simulink model "ADCS_MIL"  (R2024a)
settings: Solver=FixedStepAuto  StartTime=0.0  StopTime=6000  RelTol=1e-3
undefined symbols (not defined in the file or in its folder): agh, attitude, Cd, dgh, Eearth, epoch, Esun, Jsc, juliandate, k_Bdot, Kd1, Kd2, Kd3, km, Kp1, Kp2, Kp3, m, m_disturb, MTQ_Swithces, NoiseStd, s, satellite, signQuat, simulator, Surf_areas, Surf_dist, Surf_normals, Surf_reflectivity, WMM2020
libraries: sharedtransform x18, aerolibconvert2 x12, SepehrMILLib x11, simulink_extras x8, aerolibsatdyn x5, aerolibutil x5, sharedutil x3, vrlib x3, aerolibtransform2 x3, aerolibgravity2 x3, matrix_library x2
(part 2 of 3)

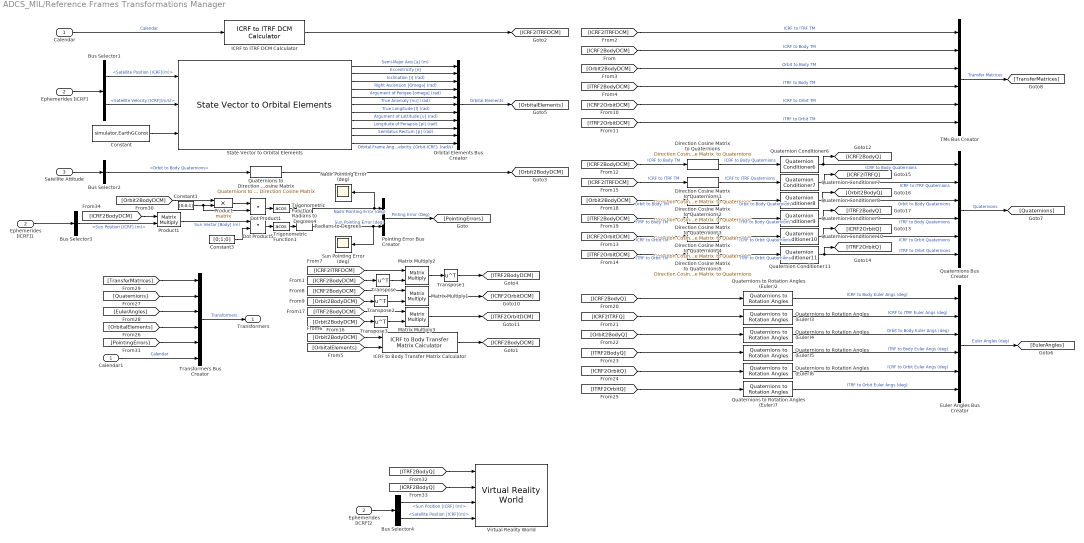
== system ADCS_MIL/Reference Frames Transformations Manager ==
  Calendar : Inport
  Ephemerides [ICRF] : Inport  Port=2
  Satellite Attitude : Inport  Port=3
  Bus Selector1 : BusSelector  OutputSignals=Satellite Ephemeris [ICRF].Satellite Position [ICRF](m),Satellite Ephemeris [ICRF].Satellite Velocity [ICRF](m/s)
  Bus Selector2 : BusSelector  OutputSignals=Orbit to Body Quaternions
  Bus Selector3 : BusSelector  OutputSignals=Sun Ephemeris [ICRF].Sun Position [ICRF] (m)
  Bus Selector4 : BusSelector  OutputSignals=Sun Ephemeris [ICRF].Sun Position [ICRF] (m),Satellite Ephemeris [ICRF].Satellite Position [ICRF](m)
  Calendar1 : InportShadow
  Constant : Constant  Value=simulator.EarthGConst
  Constant1 : Constant  Value=[0;0;1]
  Constant3 : Constant  Value=[0;1;0]
  Direction Cosine Matrix to Quaternions{,1..5} (6 alike) : sharedtransform/Direction Cosine Matrix  to Quaternions  aMode=0  action=None  tolerance=eps(2)
  Dot Product1 : DotProduct  OutDataTypeStr=Inherit: Inherit via internal rule
  Dot Product5 : DotProduct  OutDataTypeStr=Inherit: Inherit via internal rule
  Ephemerides [ICRF]1 : InportShadow  Port=2
  Ephemerides [ICRF]2 : InportShadow  Port=2
  Euler Angles Bus Creator : BusCreator  Inputs=6
  ICRF to Body Transfer Matrix Calculator : SepehrMILLib/Reference Frames Transformations Manager/ICRF to Body Transfer Matrix Calculator  SystemSampleTime=-1  VariantActivationTime=update diagram  AllowFlexibleInterface=on  Latency=0  AutoFrameSizeCalculation=off
  ICRF to ITRF DCM Calculator : SepehrMILLib/Reference Frames Transformations Manager/ICRF to ITRF DCM Calculator  SystemSampleTime=-1  VariantActivationTime=update diagram  AllowFlexibleInterface=on  Latency=0  AutoFrameSizeCalculation=off
  Matrix Multiply1 : Product  Multiplication=Matrix(*)
  Matrix Multiply2 : Product  Multiplication=Matrix(*)
  Matrix Multiply3 : Product  Multiplication=Matrix(*)
  Nadir Pointing Error (deg) : Scope
  Orbital Elements Bus Creator : BusCreator  Inputs=11
  Pointing Error Bus Creator : BusCreator  Inputs=2
  Product : Product  Multiplication=Matrix(*)
  Product1 : Product  Multiplication=Matrix(*)
  Quaternion Conditioner10 : SepehrMILLib/Reference Frames Transformations Manager/Quaternion Conditioner10  SystemSampleTime=-1  VariantActivationTime=update diagram  AllowFlexibleInterface=on  Latency=0  AutoFrameSizeCalculation=off
  Quaternion Conditioner11 : SepehrMILLib/Reference Frames Transformations Manager/Quaternion Conditioner11  SystemSampleTime=-1  VariantActivationTime=update diagram  AllowFlexibleInterface=on  Latency=0  AutoFrameSizeCalculation=off
  Quaternion Conditioner6 : SepehrMILLib/Reference Frames Transformations Manager/Quaternion Conditioner6  SystemSampleTime=-1  VariantActivationTime=update diagram  AllowFlexibleInterface=on  Latency=0  AutoFrameSizeCalculation=off
  Quaternion Conditioner7 : SepehrMILLib/Reference Frames Transformations Manager/Quaternion Conditioner7  SystemSampleTime=-1  VariantActivationTime=update diagram  AllowFlexibleInterface=on  Latency=0  AutoFrameSizeCalculation=off
  Quaternion Conditioner8 : SepehrMILLib/Reference Frames Transformations Manager/Quaternion Conditioner8  SystemSampleTime=-1  VariantActivationTime=update diagram  AllowFlexibleInterface=on  Latency=0  AutoFrameSizeCalculation=off
  Quaternion Conditioner9 : SepehrMILLib/Reference Frames Transformations Manager/Quaternion Conditioner9  SystemSampleTime=-1  VariantActivationTime=update diagram  AllowFlexibleInterface=on  Latency=0  AutoFrameSizeCalculation=off
  Quaternions Bus Creator : BusCreator  Inputs=6
  Quaternions to Direction Cosine Matrix : sharedtransform/Quaternions to  Direction Cosine Matrix  aMode=aMode
  Quaternions to Rotation Angles (Euler){2..7} (6 alike) : sharedtransform/Quaternions to Rotation Angles  rotationOrder=XYZ  aMode=aMode
  Radians to Degrees : simulink_extras/Transformations/Radians to Degrees
  Radians to Degrees4 : simulink_extras/Transformations/Radians to Degrees
  State Vector to Orbital Elements : SepehrMILLib/Reference Frames Transformations Manager/State Vector to Orbital Elements  SystemSampleTime=-1  VariantActivationTime=update diagram  AllowFlexibleInterface=on  Latency=0  AutoFrameSizeCalculation=off
  Sun Pointing Error (deg) : Scope
  TMs Bus Creator : BusCreator  Inputs=6
  Transformers Bus Creator : BusCreator  Inputs=6
  Transpose{,1..3} (4 alike) : Math  Operator=transpose
  Trigonometric Function : Trigonometry  Operator=acos
  Trigonometric Function1 : Trigonometry  Operator=acos  OutputSignalType=real
  Virtual Reality World : SepehrMILLib/Reference Frames Transformations Manager/Virtual Reality World  SystemSampleTime=-1  VariantControl=visSL3D  VariantActivationTime=update diagram  AllowFlexibleInterface=on  Latency=0  AutoFrameSizeCalculation=off
  Transformers : Outport
  wires:
  State Vector to Orbital Elements/7 -> Orbital Elements Bus Creator/7  "True Longitude [l] (rad)"
  Quaternion Conditioner8/1 -> Quaternions Bus Creator/3, [Orbit2BodyQ]  "Orbit to Body Quaternions"
  [Orbit2BodyQ] -> Quaternions to Rotation Angles (Euler)4/1
  [ITRF2OrbitQ] -> Quaternions to Rotation Angles (Euler)7/1
  [ITRF2OrbitDCM] -> Direction Cosine Matrix to Quaternions5/1  "ITRF to Orbit TM"
  Bus Selector1/2 -> State Vector to Orbital Elements/2  "<Satellite Velocity [ICRF](m/s)>"
  [ICRF2ITRFQ] -> Quaternions to Rotation Angles (Euler)3/1
  [Orbit2BodyDCM] -> Transpose3/1
  [ICRF2OrbitQ] -> Quaternions to Rotation Angles (Euler)6/1
  [ICRF2BodyDCM] -> Matrix Multiply1/1
  [EulerAngles] -> Transformers Bus Creator/3
  State Vector to Orbital Elements/6 -> Orbital Elements Bus Creator/6  "True Anomaly [nu] (rad)"
  State Vector to Orbital Elements/5 -> Orbital Elements Bus Creator/5  "Argument of Perigee [omega] (rad)"
  Bus Selector4/1 -> Virtual Reality World/3  "<Sun Position [ICRF] (m)>"
  Transformers Bus Creator/1 -> Transformers/1  "Transformers"
  State Vector to Orbital Elements/4 -> Orbital Elements Bus Creator/4  "Right Ascension [Omega] (rad)"
  State Vector to Orbital Elements/10 -> Orbital Elements Bus Creator/10  "Semilatus Rectum [p] (rad)"
  State Vector to Orbital Elements/9 -> Orbital Elements Bus Creator/9  "Longitude of Periapsis [pi] (rad)"
  Quaternion Conditioner10/1 -> Quaternions Bus Creator/5, [ICRF2OrbitQ]  "ICRF to Orbit Quaternions"
  State Vector to Orbital Elements/8 -> Orbital Elements Bus Creator/8  "Argument of Lattitude [u] (rad)"
  Quaternions to Direction Cosine Matrix/1 -> [Orbit2BodyDCM]
  State Vector to Orbital Elements/1 -> Orbital Elements Bus Creator/1  "Semi-Major Axis [a] (m)"
  [OrbitalElements] -> ICRF to Body Transfer Matrix Calculator/2
  Ephemerides [ICRF]1/1 -> Bus Selector3/1
  Dot Product5/1 -> Trigonometric Function1/1
  [ICRF2BodyDCM] -> Transpose/1
  Matrix Multiply2/1 -> Transpose1/1
  [ITRF2BodyQ] -> Virtual Reality World/1
  Bus Selector1/1 -> State Vector to Orbital Elements/1  "<Satellite Position [ICRF](m)>"
  ICRF to Body Transfer Matrix Calculator/1 -> [ICRF2BodyDCM]
  Transpose2/1 -> Matrix Multiply1/2
  ICRF to ITRF DCM Calculator/1 -> [ICRF2ITRFDCM]
  Orbital Elements Bus Creator/1 -> [OrbitalElements]  "Orbital Elements"
  Transpose1/1 -> [ITRF2BodyDCM]
  Trigonometric Function/1 -> Radians to Degrees4/1
  Matrix Multiply3/1 -> [ITRF2OrbitDCM]
  Constant3/1 -> Dot Product5/2
  [OrbitalElements] -> Transformers Bus Creator/4
  [ITRF2BodyDCM] -> Matrix Multiply3/1
  Transpose3/1 -> Matrix Multiply3/2
  Radians to Degrees4/1 -> Pointing Error Bus Creator/1, Nadir Pointing Error (deg)/1  "Nadir Pointing Error (deg)"
  Radians to Degrees/1 -> Sun Pointing Error (deg)/1, Pointing Error Bus Creator/2  "Sun Pointing Error (deg)"
  Calendar/1 -> ICRF to ITRF DCM Calculator/1  "Calendar"
  Bus Selector4/2 -> Virtual Reality World/4  "<Satellite Position [ICRF](m)>"
  Pointing Error Bus Creator/1 -> [PointingErrors]  "Pinting Error (Deg)"
  [ICRF2BodyQ] -> Virtual Reality World/2
  State Vector to Orbital Elements/11 -> Orbital Elements Bus Creator/11  "Orbital Frame Angular Velocity {Orbit-ICRF} (rad/s)"
  Constant/1 -> State Vector to Orbital Elements/3
  [Orbit2BodyDCM] -> Direction Cosine Matrix to Quaternions2/1  "Orbit to Body TM"
  [ICRF2ITRFDCM] -> TMs Bus Creator/1  "ICRF to ITRF TM"
  [ICRF2BodyDCM] -> TMs Bus Creator/2  "ICRF to Body TM"
  [PointingErrors] -> Transformers Bus Creator/5
  Transpose/1 -> Matrix Multiply2/2
  [Orbit2BodyDCM] -> Product/1
  Direction Cosine Matrix to Quaternions/1 -> Quaternion Conditioner6/1  "ICRF to Body Quaternions"
  [ICRF2OrbitDCM] -> TMs Bus Creator/5  "ICRF to Orbit TM"
  Quaternion Conditioner11/1 -> Quaternions Bus Creator/6, [ITRF2OrbitQ]  "ITRF to Orbit Quaternions"
  Direction Cosine Matrix to Quaternions3/1 -> Quaternion Conditioner9/1  "ITRF to Body Quaternions"
  [ICRF2BodyQ] -> Quaternions to Rotation Angles (Euler)2/1
  Constant1/1 -> Product/2, Dot Product1/2
  [ITRF2BodyDCM] -> TMs Bus Creator/4  "ITRF to Body TM"
  Quaternions to Rotation Angles (Euler)7/1 -> Euler Angles Bus Creator/6  "ITRF to Orbit Euler Angs (deg)"
  [Quaternions] -> Transformers Bus Creator/2
  [ITRF2OrbitDCM] -> TMs Bus Creator/6  "ITRF to Orbit TM"
  [ICRF2ITRFDCM] -> Matrix Multiply2/1
  Satellite Attitude/1 -> Bus Selector2/1
  Calendar1/1 -> Transformers Bus Creator/6  "Calendar"
  State Vector to Orbital Elements/2 -> Orbital Elements Bus Creator/2  "Eccentricity [e]"
  Quaternion Conditioner7/1 -> Quaternions Bus Creator/2, [ICRF2ITRFQ]  "ICRF to ITRF Quaternions"
  Ephemerides [ICRF]/1 -> Bus Selector1/1
  Quaternions Bus Creator/1 -> [Quaternions]  "Quaternions"
  [ICRF2ITRFDCM] -> Direction Cosine Matrix to Quaternions1/1  "ICRF to ITRF TM"
  Matrix Multiply1/1 -> [ICRF2OrbitDCM]
  Ephemerides [ICRF]2/1 -> Bus Selector4/1
  Direction Cosine Matrix to Quaternions5/1 -> Quaternion Conditioner11/1  "ITRF to Orbit Quaternions"
  Direction Cosine Matrix to Quaternions4/1 -> Quaternion Conditioner10/1  "ICRF to Orbit Quaternions"
  TMs Bus Creator/1 -> [TransferMatrices]  "Transfer Matrices"
  [ITRF2BodyDCM] -> Direction Cosine Matrix to Quaternions3/1  "ITRF to Body TM"
  Product1/1 -> Dot Product5/1  "Sun Vector [Body] (m)"
  Product/1 -> Dot Product1/1
  Bus Selector2/1 -> Quaternions to Direction Cosine Matrix/1  "<Orbit to Body Quaternions>"
  [Orbit2BodyDCM] -> Transpose2/1
  Quaternion Conditioner9/1 -> Quaternions Bus Creator/4, [ITRF2BodyQ]  "ITRF to Body Quaternions"
  Direction Cosine Matrix to Quaternions2/1 -> Quaternion Conditioner8/1  "Orbit to Body Quaternions"
  Quaternion Conditioner6/1 -> Quaternions Bus Creator/1, [ICRF2BodyQ]  "ICRF to Body Quaternions"
  Quaternions to Rotation Angles (Euler)5/1 -> Euler Angles Bus Creator/4  "ITRF to Body Euler Angs (deg)"
  Dot Product1/1 -> Trigonometric Function/1
  Direction Cosine Matrix to Quaternions1/1 -> Quaternion Conditioner7/1  "ICRF to ITRF Quaternions"
  Quaternions to Rotation Angles (Euler)2/1 -> Euler Angles Bus Creator/1  "ICRF to Body Euler Angs (deg)"
  Quaternions to Rotation Angles (Euler)3/1 -> Euler Angles Bus Creator/2  "ICRF to ITRF Euler Angs (deg)"
  Euler Angles Bus Creator/1 -> [EulerAngles]  "Euler Angles (deg)"
  State Vector to Orbital Elements/3 -> Orbital Elements Bus Creator/3  "Inclination [i] (rad)"
  [TransferMatrices] -> Transformers Bus Creator/1
  [ICRF2OrbitDCM] -> Direction Cosine Matrix to Quaternions4/1  "ICRF to Orbit TM"
  Quaternions to Rotation Angles (Euler)6/1 -> Euler Angles Bus Creator/5  "ICRF to Orbit Euler Angs (deg)"
  [ITRF2BodyQ] -> Quaternions to Rotation Angles (Euler)5/1
  [Orbit2BodyDCM] -> TMs Bus Creator/3  "Orbit to Body TM"
  Trigonometric Function1/1 -> Radians to Degrees/1
  Quaternions to Rotation Angles (Euler)4/1 -> Euler Angles Bus Creator/3  "Orbit to Body Euler Angs (deg)"
  [ICRF2BodyDCM] -> Direction Cosine Matrix to Quaternions/1  "ICRF to Body TM"
  [Orbit2BodyDCM] -> ICRF to Body Transfer Matrix Calculator/1
  [ICRF2BodyDCM] -> Product1/1
  Bus Selector3/1 -> Product1/2  "<Sun Position [ICRF] (m)>"

== system ADCS_MIL/Satellite Position [ICRF2ITRF] ==
  Satellite Position [ICRF] : Inport
  Onboard Calendar : Inport  Port=2
  Bus Selector : BusSelector  OutputSignals=Onboard Satellite Position [ICRF] (m)
  ICRF to ITRF DCM Calculator : SepehrMILLib/Reference Frames Transformations Manager/ICRF to ITRF DCM Calculator  SystemSampleTime=-1  VariantActivationTime=update diagram  AllowFlexibleInterface=on  Latency=0  AutoFrameSizeCalculation=off
  Product1 : Product  Multiplication=Matrix(*)
  Satellite Position [ITRF] (m) : Outport
  wires:
  ICRF to ITRF DCM Calculator/1 -> [ICRF2ITRFDCM]
  Onboard Calendar/1 -> ICRF to ITRF DCM Calculator/1  "Calendar"
  [ICRF2ITRFDCM] -> Product1/1
  Satellite Position [ICRF]/1 -> Bus Selector/1
  Product1/1 -> Satellite Position [ITRF] (m)/1  "Onboard_Satellite Position [ITRF] (m)"
  Bus Selector/1 -> Product1/2  "<Onboard Satellite Position [ICRF] (m)>"

== system ADCS_MIL/Sensors ==
  Calendar : Inport
  Satellite Ephemeris : Inport  Port=2
  Satellite Attitude : Inport  Port=3
  Sensor Switch : Inport  Port=4
  MM_Temp : Inport  Port=5
  Measurement Model DCM : Inport  Port=6
  Eclipse : Inport  Port=7
  Input Voltage(V) : Inport  Port=8
  B_Body : Inport  Port=9
  Sun Ephemeris [ICRF] : Inport  Port=10
  Transformers : Inport  Port=11
  Bus Creator : BusCreator  Inputs=3
  Bus Selector : BusSelector  OutputSignals=Angular Velocity {Body-ICRF}(rad/s)
  Bus Selector1 : BusSelector  OutputSignals=Sun Position [ICRF] (m)
  Bus Selector2 : BusSelector  OutputSignals=Quaternions.ICRF to Body Quaternions
  GNSS Receiver Model : Subsystem
  Gyroscope Model : Subsystem
  Magnetometer Model : Subsystem
  Sun Sensor Model : Subsystem
  Sun Position Measured [Body] : Outport
  B Measured [Body] : Outport  Port=2
  Angular Velocity Measured [Body] : Outport  Port=3
  Satellite Measured Ephemeris : Outport  Port=4
  Current (A) : Outport  Port=5
  wires:
  Calendar/1 -> GNSS Receiver Model/1(Calendar)
  Satellite Ephemeris/1 -> GNSS Receiver Model/2(Satellite Ephemeris)
  Satellite Attitude/1 -> Bus Selector/1
  Sensor Switch/1 -> Magnetometer Model/5(Sensor Switch), GNSS Receiver Model/4(Sensor Switch), Gyroscope Model/4(Sensor Switch)
  MM_Temp/1 -> Magnetometer Model/2(Temperature (˚C))
  Input Voltage(V)/1 -> Magnetometer Model/3(Input Voltage (V)), GNSS Receiver Model/3(" Input Voltage (V)"), Gyroscope Model/2(Input Voltage (V))
  Measurement Model DCM/1 -> Gyroscope Model/3(Measurement Model DCM), Magnetometer Model/4(Measurement Model DCM)
  Eclipse/1 -> Sun Sensor Model/1(Eclipse)
  Sun Sensor Model/1(SunPos_Sensed(Body)) -> Sun Position Measured [Body]/1
  Magnetometer Model/2(Power (W)) -> Bus Creator/3  "Magnetometer Power (W)"
  Magnetometer Model/1(Magnetic Field [Sensor](T)) -> B Measured [Body]/1
  Gyroscope Model/2(Power (W)) -> Bus Creator/2  "Gyro Power (W)"
  GNSS Receiver Model/2(Power (W)) -> Bus Creator/1  "Power GNSS Receiver (W)"
  Bus Creator/1 -> Current (A)/1
  GNSS Receiver Model/1(Measured Satellite Ephemeris) -> Satellite Measured Ephemeris/1
  Gyroscope Model/1(Measured Angular Velocity [Sensor] (rad/s)) -> Angular Velocity Measured [Body]/1
  B_Body/1 -> Magnetometer Model/1(Magnetic Field [Body] (T))
  Bus Selector/1 -> Gyroscope Model/1(Angular Velocity [Body] (rad/s))  "<Angular Velocity {Body-ICRF}(rad/s)>"
  Sun Ephemeris [ICRF]/1 -> Bus Selector1/1
  Bus Selector1/1 -> Sun Sensor Model/3(SunPos[ICRF])  "<Sun Position [ICRF] (m)>"
  Transformers/1 -> Bus Selector2/1
  Bus Selector2/1 -> Sun Sensor Model/2(q[ICRFtoBody])  "<ICRF to Body Quaternions>"

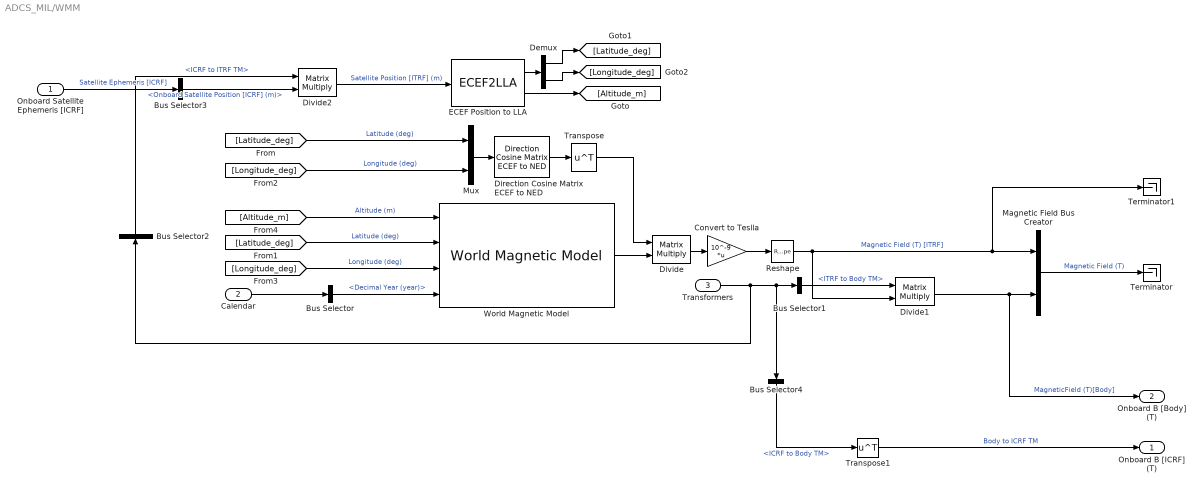
== system ADCS_MIL/WMM ==
  Onboard Satellite Ephemeris [ICRF] : Inport
  Calendar : Inport  Port=2
  Transformers : Inport  Port=3
  Bus Selector : BusSelector  OutputSignals=Decimal Year (year)
  Bus Selector1 : BusSelector  OutputSignals=Transfer Matrices.ITRF to Body TM
  Bus Selector2 : BusSelector  OutputSignals=Transfer Matrices.ICRF to ITRF TM
  Bus Selector3 : BusSelector  OutputSignals=Onboard Satellite Position [ICRF] (m)
  Bus Selector4 : BusSelector  OutputSignals=Transfer Matrices.ICRF to Body TM
  Convert to Teslla : Gain  Gain=10^-9  Multiplication=Matrix(K*u)
  Demux : Demux  Outputs=2
  Direction Cosine Matrix ECEF to NED : aerolibtransform2/Direction Cosine Matrix ECEF to NED
  Divide : Product  Inputs=**  Multiplication=Matrix(*)
  Divide1 : Product  Inputs=**  Multiplication=Matrix(*)
  Divide2 : Product  Inputs=**  Multiplication=Matrix(*)
  ECEF Position to LLA : ECEF2LLA
  Magnetic Field Bus Creator : BusCreator  Inputs=2
  Mux : Mux  Inputs=2
  Reshape : Reshape  OutputDimensionality=Customize  OutputDimensions=[3,1]
  Terminator : Terminator
  Terminator1 : Terminator
  Transpose : Math  Operator=transpose
  Transpose1 : Math  Operator=transpose
  World Magnetic Model : aerolibgravity2/World Magnetic Model  model=WMM2020 (2020-2025)  customFile='WMM2020.COF'  units=Metric (MKS)  time_in=on  month=January  day=1  year=2020  action=Error  h_out=off  dec_out=off  inc_out=off  ti_out=off
  Onboard B [ICRF] (T) : Outport
  Onboard B [Body] (T) : Outport  Port=2
  wires:
  [Latitude_deg] -> World Magnetic Model/2  "Latitude (deg)"
  Transpose/1 -> Divide/1
  Demux/1 -> [Latitude_deg]
  [Altitude_m] -> World Magnetic Model/1  "Altitude (m)"
  Reshape/1 -> Terminator1/1, Magnetic Field Bus Creator/1, Divide1/2  "Magnetic Field (T) [ITRF]"
  Direction Cosine Matrix ECEF to NED/1 -> Transpose/1
  Magnetic Field Bus Creator/1 -> Terminator/1  "Magnetic Field (T)"
  Mux/1 -> Direction Cosine Matrix ECEF to NED/1
  Transformers/1 -> Bus Selector1/1, Bus Selector4/1, Bus Selector2/1
  [Latitude_deg] -> Mux/1  "Latitude (deg)"
  [Longitude_deg] -> Mux/2  "Longitude (deg)"
  ECEF Position to LLA/2 -> [Altitude_m]
  Demux/2 -> [Longitude_deg]
  Divide/1 -> Convert to Teslla/1
  Convert to Teslla/1 -> Reshape/1
  Calendar/1 -> Bus Selector/1
  ECEF Position to LLA/1 -> Demux/1
  Divide2/1 -> ECEF Position to LLA/1  "Satellite Position [ITRF] (m)"
  [Longitude_deg] -> World Magnetic Model/3  "Longitude (deg)"
  Bus Selector/1 -> World Magnetic Model/4  "<Decimal Year (year)>"
  Divide1/1 -> Onboard B [Body] (T)/1, Magnetic Field Bus Creator/2  "MagneticField (T)[Body]"
  World Magnetic Model/1 -> Divide/2
  Bus Selector1/1 -> Divide1/1  "<ITRF to Body TM>"
  Onboard Satellite Ephemeris [ICRF]/1 -> Bus Selector3/1  "Satellite Ephemeris [ICRF]"
  Bus Selector2/1 -> Divide2/1  "<ICRF to ITRF TM>"
  Bus Selector3/1 -> Divide2/2  "<Onboard Satellite Position [ICRF] (m)>"
  Bus Selector4/1 -> Transpose1/1  "<ICRF to Body TM>"
  Transpose1/1 -> Onboard B [ICRF] (T)/1  "Body to ICRF TM"

== system ADCS_MIL/Attitude Controlgg/On.Nadir_Pointing/Nadir Pointing ==
  Ephemeris : Inport
  q(body2ICRF) : Inport  Port=2
  Omega(Body) : Inport  Port=3
  B(Body) : Inport  Port=4
  Kd : Constant  Value=[1 1 1]
  Kp : Constant  Value=[1 1 1]
  PD Controller : Subsystem
  q_Desired Propagator : Subsystem
  q_error Calculator : Subsystem
  m_Command : Outport
  wires:
  q(body2ICRF)/1 -> q_error Calculator/2(q_Real)
  Ephemeris/1 -> q_Desired Propagator/1(Ephemeris)
  q_Desired Propagator/1(q_Desired) -> q_error Calculator/1(q_Desired)
  PD Controller/1(m_Command) -> m_Command/1
  q_error Calculator/1(q_error) -> PD Controller/3(q_Error)
  Kp/1 -> PD Controller/4(Kp)
  Kd/1 -> PD Controller/5(Kd)
  Omega(Body)/1 -> PD Controller/1(Omega(Body))
  B(Body)/1 -> PD Controller/2(B(Body))

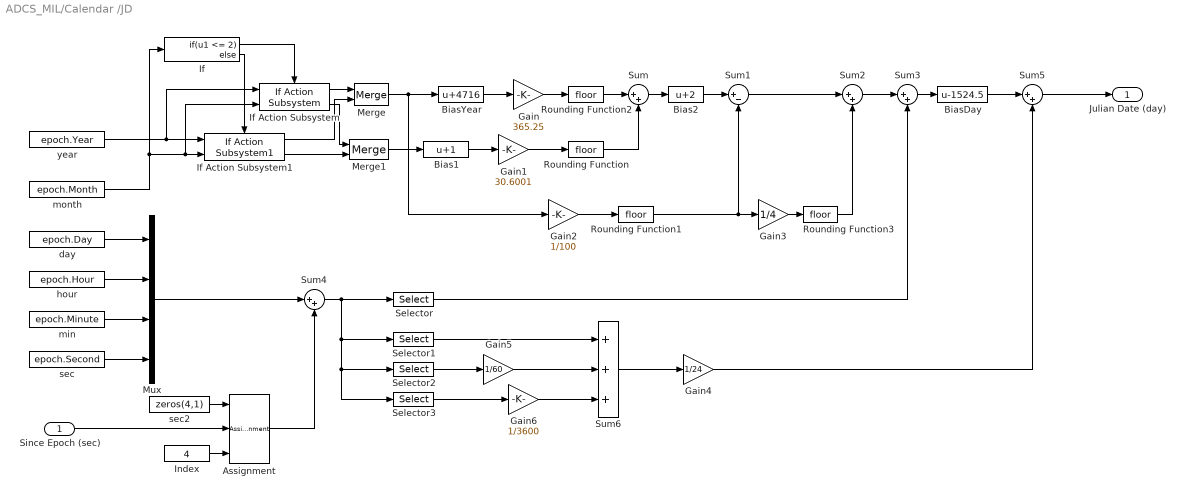
== system ADCS_MIL/Calendar /JD ==
  Since Epoch (sec) : Inport  OutMin=0  PortDimensions=1
  Assignment : Assignment  IndexOptions=Index vector (port)  Indices=1  OutputSizes=1
  Bias1 : Bias  Bias=1  SaturateOnIntegerOverflow=off
  Bias2 : Bias  Bias=2  SaturateOnIntegerOverflow=off
  BiasDay : Bias  Bias=-1524.5  SaturateOnIntegerOverflow=off
  BiasYear : Bias  Bias=4716  SaturateOnIntegerOverflow=off
  Gain : Gain  Gain=365.25
  Gain1 : Gain  Gain=30.6001
  Gain2 : Gain  Gain=1/100
  Gain3 : Gain  Gain=1/4
  Gain4 : Gain  Gain=1/24
  Gain5 : Gain  Gain=1/60
  Gain6 : Gain  Gain=1/3600
  If : If  IfExpression=u1 <= 2
  If Action Subsystem : aerolibconvert2/Julian Date Conversion/If Action Subsystem  SystemSampleTime=-1  VariantActivationTime=update diagram  AllowFlexibleInterface=on  Latency=0  AutoFrameSizeCalculation=off
  If Action Subsystem1 : aerolibconvert2/Julian Date Conversion/If Action Subsystem1  SystemSampleTime=-1  VariantActivationTime=update diagram  AllowFlexibleInterface=on  Latency=0  AutoFrameSizeCalculation=off
  Index : Constant  Value=4
  Merge : Merge
  Merge1 : Merge
  Mux : Mux
  Rounding Function{,1..3} (4 alike) : Rounding
  Selector : Selector  InputPortWidth=4  IndexOptions=Index vector (dialog)  Indices=[1]  OutputSizes=1
  Selector1 : Selector  InputPortWidth=4  IndexOptions=Index vector (dialog)  Indices=[2]  OutputSizes=1
  Selector2 : Selector  InputPortWidth=4  IndexOptions=Index vector (dialog)  Indices=[3]  OutputSizes=1
  Selector3 : Selector  InputPortWidth=4  IndexOptions=Index vector (dialog)  Indices=[4]  OutputSizes=1
  Sum{,2..5} (5 alike) : Sum  Inputs=|++
  Sum1 : Sum  Inputs=|+-
  Sum6 : Sum  Inputs=+++
  day : Constant  Value=epoch.Day
  hour : Constant  Value=epoch.Hour
  min : Constant  Value=epoch.Minute
  month : Constant  Value=epoch.Month
  sec : Constant  Value=epoch.Second
  sec2 : Constant  Value=zeros(4,1)
  year : Constant  Value=epoch.Year
  Julian Date (day) : Outport  VectorParamsAs1DForOutWhenUnconnected=off
  wires:
  Merge1/1 -> Bias1/1
  Mux/1 -> Sum4/1
  month/1 -> If/1, If Action Subsystem1/2, If Action Subsystem/2
  Rounding Function/1 -> Sum/2
  day/1 -> Mux/1
  If Action Subsystem1/2 -> Merge1/2
  Sum/1 -> Bias2/1
  Sum6/1 -> Gain4/1
  BiasDay/1 -> Sum5/1
  hour/1 -> Mux/2
  Selector/1 -> Sum3/2
  sec/1 -> Mux/4
  Since Epoch (sec)/1 -> Assignment/2
  If/2 -> If Action Subsystem1/Action
  Rounding Function1/1 -> Sum1/2, Gain3/1
  Gain5/1 -> Sum6/2
  Assignment/1 -> Sum4/2
  Bias2/1 -> Sum1/1
  Gain/1 -> Rounding Function2/1
  Gain2/1 -> Rounding Function1/1
  Sum4/1 -> Selector/1, Selector3/1, Selector2/1, Selector1/1
  If Action Subsystem/1 -> Merge/1
  year/1 -> If Action Subsystem1/1, If Action Subsystem/1
  Gain6/1 -> Sum6/3
  Sum3/1 -> BiasDay/1
  If Action Subsystem/2 -> Merge1/1
  Bias1/1 -> Gain1/1
  Rounding Function3/1 -> Sum2/2
  Gain1/1 -> Rounding Function/1
  sec2/1 -> Assignment/1
  Sum1/1 -> Sum2/1
  Sum5/1 -> Julian Date (day)/1
  Selector1/1 -> Sum6/1
  Sum2/1 -> Sum3/1
  Gain4/1 -> Sum5/2
  BiasYear/1 -> Gain/1
  Merge/1 -> BiasYear/1, Gain2/1
  Gain3/1 -> Rounding Function3/1
  Selector2/1 -> Gain5/1
  Rounding Function2/1 -> Sum/1
  Selector3/1 -> Gain6/1
  If/1 -> If Action Subsystem/Action
  min/1 -> Mux/3
  If Action Subsystem1/1 -> Merge/2
  Index/1 -> Assignment/3

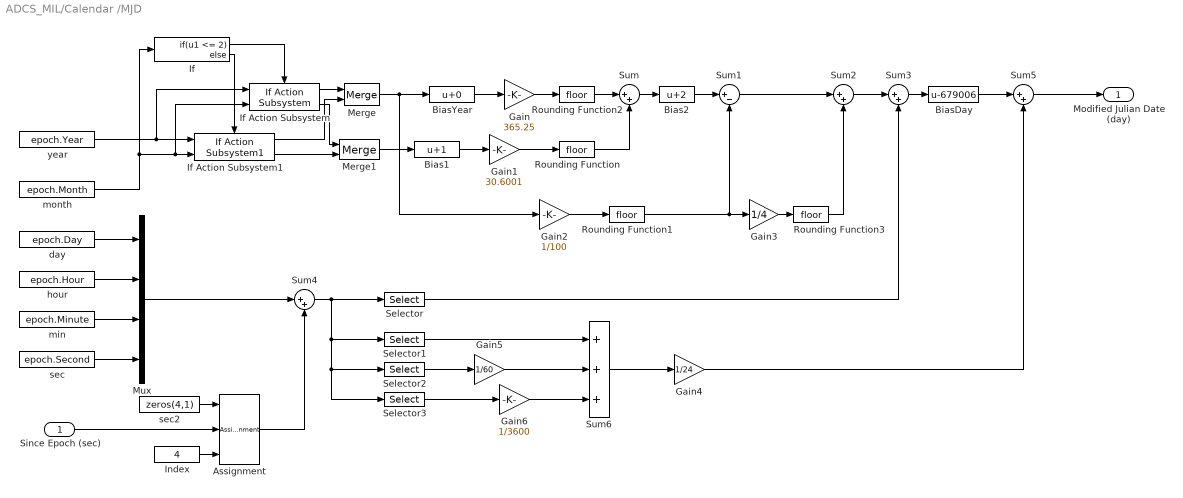
== system ADCS_MIL/Calendar /MJD ==
  Since Epoch (sec) : Inport  OutMin=0  PortDimensions=1
  Assignment : Assignment  IndexOptions=Index vector (port)  Indices=1  OutputSizes=1
  Bias1 : Bias  Bias=1  SaturateOnIntegerOverflow=off
  Bias2 : Bias  Bias=2  SaturateOnIntegerOverflow=off
  BiasDay : Bias  Bias=-679006  SaturateOnIntegerOverflow=off
  BiasYear : Bias  SaturateOnIntegerOverflow=off
  Gain : Gain  Gain=365.25
  Gain1 : Gain  Gain=30.6001
  Gain2 : Gain  Gain=1/100
  Gain3 : Gain  Gain=1/4
  Gain4 : Gain  Gain=1/24
  Gain5 : Gain  Gain=1/60
  Gain6 : Gain  Gain=1/3600
  If : If  IfExpression=u1 <= 2
  If Action Subsystem : aerolibconvert2/Julian Date Conversion/If Action Subsystem  SystemSampleTime=-1  VariantActivationTime=update diagram  AllowFlexibleInterface=on  Latency=0  AutoFrameSizeCalculation=off
  If Action Subsystem1 : aerolibconvert2/Julian Date Conversion/If Action Subsystem1  SystemSampleTime=-1  VariantActivationTime=update diagram  AllowFlexibleInterface=on  Latency=0  AutoFrameSizeCalculation=off
  Index : Constant  Value=4
  Merge : Merge
  Merge1 : Merge
  Mux : Mux
  Rounding Function{,1..3} (4 alike) : Rounding
  Selector : Selector  InputPortWidth=4  IndexOptions=Index vector (dialog)  Indices=[1]  OutputSizes=1
  Selector1 : Selector  InputPortWidth=4  IndexOptions=Index vector (dialog)  Indices=[2]  OutputSizes=1
  Selector2 : Selector  InputPortWidth=4  IndexOptions=Index vector (dialog)  Indices=[3]  OutputSizes=1
  Selector3 : Selector  InputPortWidth=4  IndexOptions=Index vector (dialog)  Indices=[4]  OutputSizes=1
  Sum{,2..5} (5 alike) : Sum  Inputs=|++
  Sum1 : Sum  Inputs=|+-
  Sum6 : Sum  Inputs=+++
  day : Constant  Value=epoch.Day
  hour : Constant  Value=epoch.Hour
  min : Constant  Value=epoch.Minute
  month : Constant  Value=epoch.Month
  sec : Constant  Value=epoch.Second
  sec2 : Constant  Value=zeros(4,1)
  year : Constant  Value=epoch.Year
  Modified Julian Date (day) : Outport  VectorParamsAs1DForOutWhenUnconnected=off
  wires:
  Rounding Function/1 -> Sum/2
  If/2 -> If Action Subsystem1/Action
  Gain4/1 -> Sum5/2
  BiasYear/1 -> Gain/1
  Bias2/1 -> Sum1/1
  Selector1/1 -> Sum6/1
  Sum/1 -> Bias2/1
  Sum2/1 -> Sum3/1
  BiasDay/1 -> Sum5/1
  Selector/1 -> Sum3/2
  Sum1/1 -> Sum2/1
  year/1 -> If Action Subsystem1/1, If Action Subsystem/1
  Sum5/1 -> Modified Julian Date (day)/1
  Sum6/1 -> Gain4/1
  hour/1 -> Mux/2
  Gain/1 -> Rounding Function2/1
  Merge1/1 -> Bias1/1
  Since Epoch (sec)/1 -> Assignment/2
  Gain6/1 -> Sum6/3
  Gain2/1 -> Rounding Function1/1
  Mux/1 -> Sum4/1
  Rounding Function1/1 -> Sum1/2, Gain3/1
  Rounding Function3/1 -> Sum2/2
  Sum3/1 -> BiasDay/1
  Selector3/1 -> Gain6/1
  Rounding Function2/1 -> Sum/1
  Gain1/1 -> Rounding Function/1
  sec2/1 -> Assignment/1
  day/1 -> Mux/1
  Bias1/1 -> Gain1/1
  min/1 -> Mux/3
  Gain3/1 -> Rounding Function3/1
  If/1 -> If Action Subsystem/Action
  Gain5/1 -> Sum6/2
  If Action Subsystem1/1 -> Merge/2
  Sum4/1 -> Selector/1, Selector3/1, Selector2/1, Selector1/1
  Merge/1 -> BiasYear/1, Gain2/1
  If Action Subsystem/1 -> Merge/1
  Selector2/1 -> Gain5/1
  If Action Subsystem/2 -> Merge1/1
  month/1 -> If/1, If Action Subsystem1/2, If Action Subsystem/2
  sec/1 -> Mux/4
  If Action Subsystem1/2 -> Merge1/2
  Assignment/1 -> Sum4/2
  Index/1 -> Assignment/3

== system ADCS_MIL/External Disturbance Torque/Drag ==
  Rsc_earth : Inport
  Vsc_earth : Inport  Port=2
  Abn : Inport  Port=3
  Constant : Constant  Value=Surf_normals
  Constant1 : Constant  Value=Surf_areas
  Constant2 : Constant  Value=Cd
  Constant4 : Constant  Value=Surf_dist
  MATLAB Function : MATLAB Function  TreatAsAtomicUnit=on
  Drag torque : Outport
  wires:
  Abn/1 -> MATLAB Function/3(Abn)
  Rsc_earth/1 -> MATLAB Function/1(Rearth)
  MATLAB Function/1(M_drag) -> Drag torque/1
  Constant/1 -> MATLAB Function/4(Surf_norms)
  Constant1/1 -> MATLAB Function/5(Surf_areas)
  Constant4/1 -> MATLAB Function/6(Surf_dist)
  Vsc_earth/1 -> MATLAB Function/2(Vearth)
  Constant2/1 -> MATLAB Function/7(Cd)

== system ADCS_MIL/External Disturbance Torque/Gravitional ==
  Rsc_earth : Inport
  Vsc_earth : Inport  Port=2
  Abn : Inport  Port=3
  Constant : Constant  Value=Jsc
  MATLAB Function : MATLAB Function  TreatAsAtomicUnit=on
  Grav torque : Outport
  wires:
  Abn/1 -> MATLAB Function/3(Abn)
  Rsc_earth/1 -> MATLAB Function/1(Rearth)
  MATLAB Function/1(M_grav) -> Grav torque/1
  Constant/1 -> MATLAB Function/4(J)
  Vsc_earth/1 -> MATLAB Function/2(Vearth)

== system ADCS_MIL/External Disturbance Torque/Magnetic ==
  Rsc_earth : Inport
  Earth RA : Inport  Port=2
  Abn : Inport  Port=3
  Att_req_inert1 : MATLAB Function  TreatAsAtomicUnit=on
  Constant : Constant  Value=agh
  Constant1 : Constant  Value=m_disturb
  Constant3 : Constant  Value=dgh
  Cross Product : vrlib/Utilities/Cross Product
  Magnetic Disturbance Torques Calculator : MATLAB Function  TreatAsAtomicUnit=on
  Product : Product  Multiplication=Matrix(*)
  Bn : Outport
  Bb : Outport  Port=2
  Magnetic torque : Outport  Port=3
  wires:
  Att_req_inert1/1(Bn) -> Product/2, Bn/1
  Rsc_earth/1 -> Att_req_inert1/3(R)
  Constant3/1 -> Att_req_inert1/1(dgh)
  Constant/1 -> Att_req_inert1/2(agh)
  Earth RA/1 -> Att_req_inert1/4(RA_earth_rot)
  Abn/1 -> Product/1
  Product/1 -> Cross Product/1, Bb/1
  Constant1/1 -> Cross Product/2
  Cross Product/1 -> Magnetic torque/1

== system ADCS_MIL/External Disturbance Torque/Radiation Pressure ==
  Rsc_sun : Inport
  Rsc_earth : Inport  Port=2
  Abn : Inport  Port=3
  Constant : Constant  Value=Surf_normals
  Constant1 : Constant  Value=Surf_areas
  Constant2 : Constant  Value=Surf_reflectivity
  Constant3 : Constant  Value=Esun
  Constant4 : Constant  Value=Surf_dist
  Constant5 : Constant  Value=Eearth
  MATLAB Function : MATLAB Function  TreatAsAtomicUnit=on
  MATLAB Function1 : MATLAB Function  TreatAsAtomicUnit=on
  Scope : Scope  NumInputPorts=2
  Sum : Sum
  RP torque : Outport
  wires:
  Abn/1 -> MATLAB Function1/2(Abn), MATLAB Function/2(Abn)
  Rsc_sun/1 -> MATLAB Function/1(Rsun)
  MATLAB Function/1(M_srp) -> Scope/1, Sum/1
  Constant/1 -> MATLAB Function1/3(Surf_norms), MATLAB Function/3(Surf_norms)
  Constant1/1 -> MATLAB Function1/4(Surf_areas), MATLAB Function/4(Surf_areas)
  Constant2/1 -> MATLAB Function1/5(Surf_reflec), MATLAB Function/5(Surf_reflec)
  Constant3/1 -> MATLAB Function/7(Esun)
  Constant4/1 -> MATLAB Function1/6(Surf_dist), MATLAB Function/6(Surf_dist)
  Sum/1 -> RP torque/1
  MATLAB Function1/1(M_srp) -> Sum/2, Scope/2
  Rsc_earth/1 -> MATLAB Function1/1(R)
  Constant5/1 -> MATLAB Function1/7(E)

== system ADCS_MIL/Nadir Pointing Algorithm/PD Controller ==
  Omega(Body) : Inport
  B(Body) : Inport  Port=2
  q_Error : Inport  Port=3
  Kp : Inport  Port=4
  Kd : Inport  Port=5
  MATLAB Function : MATLAB Function  TreatAsAtomicUnit=on
  Saturation : Saturate  UpperLimit=5  LowerLimit=-5
  Scope : Scope
  m_Command : Outport
  wires:
  MATLAB Function/1(m_Command) -> Saturation/1
  q_Error/1 -> MATLAB Function/1(q_Error)
  Omega(Body)/1 -> MATLAB Function/2(omega_Body)
  Kp/1 -> MATLAB Function/3(Kp)
  Kd/1 -> MATLAB Function/4(Kd)
  B(Body)/1 -> MATLAB Function/5(B_body)
  Saturation/1 -> Scope/1, m_Command/1

== system ADCS_MIL/Nadir Pointing Algorithm/q_Desired Propagator ==
  Satellite Ephemeris : Inport
  q [Body2ICRF] : Inport  Port=2
  Attitude Profile (Nadir Pointing) : aerolibsatdyn/Attitude Profile (Nadir Pointing)  outputError=on  outputFinalAttitude=off  portFrame=ICRF  pointingMode=Point at nadir  celestialTarget=Sun  tunablePointing=off  primaryAlignmentSrc=Dialog  primaryAlignment=[0 0 1]  secondaryAlignmentSrc=Dialog  secondaryAlignment=[1 0 0]  constraintFrame=ICRF  primaryConstraintSrc=Dialog  primaryConstraint=[1 0 0]  secondaryConstraintSrc=Dialog  secondaryConstraint=[0 1 0]
  Bus Selector : BusSelector  OutputSignals=Onboard Satellite Position [ICRF] (m),Onboard Satellite Velocity [ICRF] (m/s)
  Bus Selector1 : BusSelector  OutputSignals=Onboard Satellite Position [ICRF] (m)
  Demux : Demux
  Demux1 : Demux
  MATLAB Function : MATLAB Function  TreatAsAtomicUnit=on
  Satellite Ephemeris1 : InportShadow
  Scope{,1..9} (10 alike) : Scope
  q_Desired : Outport
  wires:
  Satellite Ephemeris/1 -> Bus Selector/1
  Bus Selector/2 -> MATLAB Function/2(v_sat_ICRF)  "<Onboard Satellite Velocity [ICRF] (m/s)>"
  Bus Selector/1 -> MATLAB Function/1(r_sat_ICRF)  "<Onboard Satellite Position [ICRF] (m)>"
  Attitude Profile (Nadir Pointing)/1 -> Scope/1, q_Desired/1, Demux/1
  Demux/1 -> Scope1/1
  Demux/2 -> Scope2/1
  Demux/3 -> Scope3/1
  Demux/4 -> Scope4/1
  Demux1/1 -> Scope6/1
  Demux1/2 -> Scope7/1
  Demux1/4 -> Scope9/1
  Demux1/3 -> Scope8/1
  MATLAB Function/1(q_Desired) -> Demux1/1, Scope5/1
  Satellite Ephemeris1/1 -> Bus Selector1/1
  Bus Selector1/1 -> Attitude Profile (Nadir Pointing)/1  "<Onboard Satellite Position [ICRF] (m)>"
  q [Body2ICRF]/1 -> Attitude Profile (Nadir Pointing)/2

== system ADCS_MIL/Nadir Pointing Algorithm/q_error Calculator ==
  q_Desired : Inport
  q_Real : Inport  Port=2
  MATLAB Function : MATLAB Function  TreatAsAtomicUnit=on
  q_Error : Outport
  wires:
  MATLAB Function/1(q_Error) -> q_Error/1
  q_Desired/1 -> MATLAB Function/1(q_Real)
  q_Real/1 -> MATLAB Function/2(q_Desired)

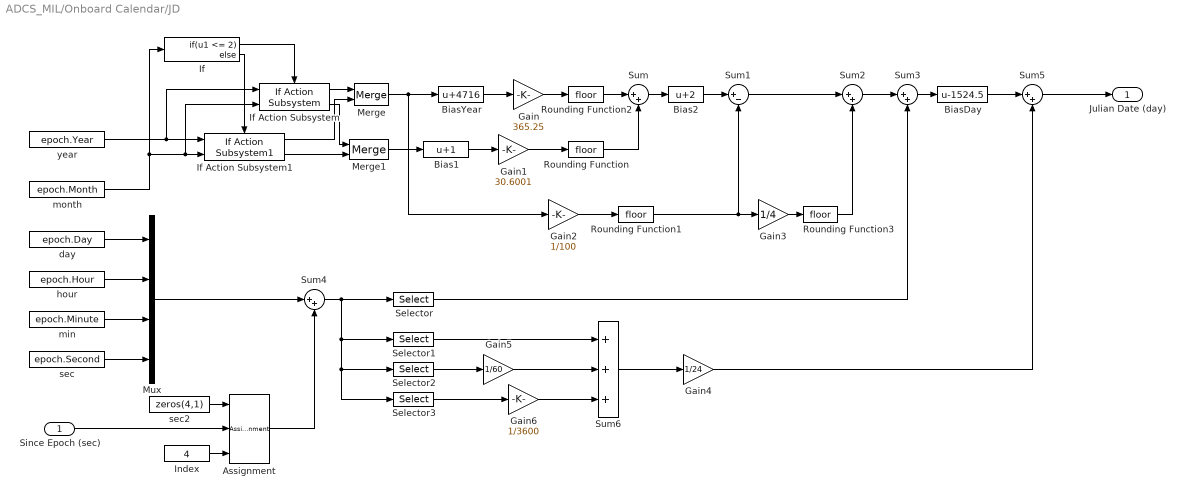
== system ADCS_MIL/Onboard Calendar/JD ==
  Since Epoch (sec) : Inport  OutMin=0  PortDimensions=1
  Assignment : Assignment  IndexOptions=Index vector (port)  Indices=1  OutputSizes=1
  Bias1 : Bias  Bias=1  SaturateOnIntegerOverflow=off
  Bias2 : Bias  Bias=2  SaturateOnIntegerOverflow=off
  BiasDay : Bias  Bias=-1524.5  SaturateOnIntegerOverflow=off
  BiasYear : Bias  Bias=4716  SaturateOnIntegerOverflow=off
  Gain : Gain  Gain=365.25
  Gain1 : Gain  Gain=30.6001
  Gain2 : Gain  Gain=1/100
  Gain3 : Gain  Gain=1/4
  Gain4 : Gain  Gain=1/24
  Gain5 : Gain  Gain=1/60
  Gain6 : Gain  Gain=1/3600
  If : If  IfExpression=u1 <= 2
  If Action Subsystem : aerolibconvert2/Julian Date Conversion/If Action Subsystem  SystemSampleTime=-1  VariantActivationTime=update diagram  AllowFlexibleInterface=on  Latency=0  AutoFrameSizeCalculation=off
  If Action Subsystem1 : aerolibconvert2/Julian Date Conversion/If Action Subsystem1  SystemSampleTime=-1  VariantActivationTime=update diagram  AllowFlexibleInterface=on  Latency=0  AutoFrameSizeCalculation=off
  Index : Constant  Value=4
  Merge : Merge
  Merge1 : Merge
  Mux : Mux
  Rounding Function{,1..3} (4 alike) : Rounding
  Selector : Selector  InputPortWidth=4  IndexOptions=Index vector (dialog)  Indices=[1]  OutputSizes=1
  Selector1 : Selector  InputPortWidth=4  IndexOptions=Index vector (dialog)  Indices=[2]  OutputSizes=1
  Selector2 : Selector  InputPortWidth=4  IndexOptions=Index vector (dialog)  Indices=[3]  OutputSizes=1
  Selector3 : Selector  InputPortWidth=4  IndexOptions=Index vector (dialog)  Indices=[4]  OutputSizes=1
  Sum{,2..5} (5 alike) : Sum  Inputs=|++
  Sum1 : Sum  Inputs=|+-
  Sum6 : Sum  Inputs=+++
  day : Constant  Value=epoch.Day
  hour : Constant  Value=epoch.Hour
  min : Constant  Value=epoch.Minute
  month : Constant  Value=epoch.Month
  sec : Constant  Value=epoch.Second
  sec2 : Constant  Value=zeros(4,1)
  year : Constant  Value=epoch.Year
  Julian Date (day) : Outport  VectorParamsAs1DForOutWhenUnconnected=off
  wires:
  Merge1/1 -> Bias1/1
  Mux/1 -> Sum4/1
  month/1 -> If/1, If Action Subsystem1/2, If Action Subsystem/2
  Rounding Function/1 -> Sum/2
  day/1 -> Mux/1
  If Action Subsystem1/2 -> Merge1/2
  Sum/1 -> Bias2/1
  Sum6/1 -> Gain4/1
  BiasDay/1 -> Sum5/1
  hour/1 -> Mux/2
  Selector/1 -> Sum3/2
  sec/1 -> Mux/4
  Since Epoch (sec)/1 -> Assignment/2
  If/2 -> If Action Subsystem1/Action
  Rounding Function1/1 -> Sum1/2, Gain3/1
  Gain5/1 -> Sum6/2
  Assignment/1 -> Sum4/2
  Bias2/1 -> Sum1/1
  Gain/1 -> Rounding Function2/1
  Gain2/1 -> Rounding Function1/1
  Sum4/1 -> Selector/1, Selector3/1, Selector2/1, Selector1/1
  If Action Subsystem/1 -> Merge/1
  year/1 -> If Action Subsystem1/1, If Action Subsystem/1
  Gain6/1 -> Sum6/3
  Sum3/1 -> BiasDay/1
  If Action Subsystem/2 -> Merge1/1
  Bias1/1 -> Gain1/1
  Rounding Function3/1 -> Sum2/2
  Gain1/1 -> Rounding Function/1
  sec2/1 -> Assignment/1
  Sum1/1 -> Sum2/1
  Sum5/1 -> Julian Date (day)/1
  Selector1/1 -> Sum6/1
  Sum2/1 -> Sum3/1
  Gain4/1 -> Sum5/2
  BiasYear/1 -> Gain/1
  Merge/1 -> BiasYear/1, Gain2/1
  Gain3/1 -> Rounding Function3/1
  Selector2/1 -> Gain5/1
  Rounding Function2/1 -> Sum/1
  Selector3/1 -> Gain6/1
  If/1 -> If Action Subsystem/Action
  min/1 -> Mux/3
  If Action Subsystem1/1 -> Merge/2
  Index/1 -> Assignment/3

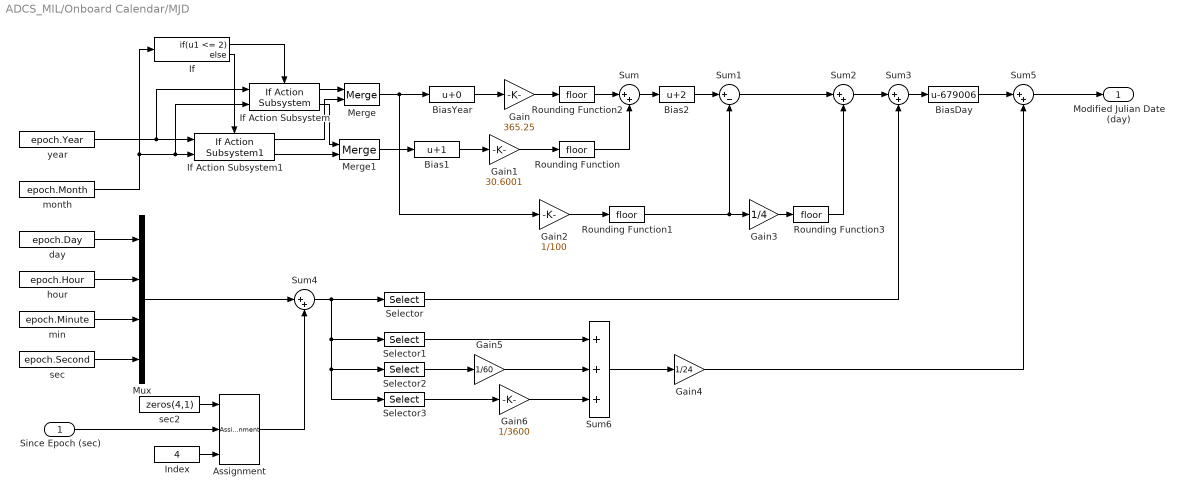
== system ADCS_MIL/Onboard Calendar/MJD ==
  Since Epoch (sec) : Inport  OutMin=0  PortDimensions=1
  Assignment : Assignment  IndexOptions=Index vector (port)  Indices=1  OutputSizes=1
  Bias1 : Bias  Bias=1  SaturateOnIntegerOverflow=off
  Bias2 : Bias  Bias=2  SaturateOnIntegerOverflow=off
  BiasDay : Bias  Bias=-679006  SaturateOnIntegerOverflow=off
  BiasYear : Bias  SaturateOnIntegerOverflow=off
  Gain : Gain  Gain=365.25
  Gain1 : Gain  Gain=30.6001
  Gain2 : Gain  Gain=1/100
  Gain3 : Gain  Gain=1/4
  Gain4 : Gain  Gain=1/24
  Gain5 : Gain  Gain=1/60
  Gain6 : Gain  Gain=1/3600
  If : If  IfExpression=u1 <= 2
  If Action Subsystem : aerolibconvert2/Julian Date Conversion/If Action Subsystem  SystemSampleTime=-1  VariantActivationTime=update diagram  AllowFlexibleInterface=on  Latency=0  AutoFrameSizeCalculation=off
  If Action Subsystem1 : aerolibconvert2/Julian Date Conversion/If Action Subsystem1  SystemSampleTime=-1  VariantActivationTime=update diagram  AllowFlexibleInterface=on  Latency=0  AutoFrameSizeCalculation=off
  Index : Constant  Value=4
  Merge : Merge
  Merge1 : Merge
  Mux : Mux
  Rounding Function{,1..3} (4 alike) : Rounding
  Selector : Selector  InputPortWidth=4  IndexOptions=Index vector (dialog)  Indices=[1]  OutputSizes=1
  Selector1 : Selector  InputPortWidth=4  IndexOptions=Index vector (dialog)  Indices=[2]  OutputSizes=1
  Selector2 : Selector  InputPortWidth=4  IndexOptions=Index vector (dialog)  Indices=[3]  OutputSizes=1
  Selector3 : Selector  InputPortWidth=4  IndexOptions=Index vector (dialog)  Indices=[4]  OutputSizes=1
  Sum{,2..5} (5 alike) : Sum  Inputs=|++
  Sum1 : Sum  Inputs=|+-
  Sum6 : Sum  Inputs=+++
  day : Constant  Value=epoch.Day
  hour : Constant  Value=epoch.Hour
  min : Constant  Value=epoch.Minute
  month : Constant  Value=epoch.Month
  sec : Constant  Value=epoch.Second
  sec2 : Constant  Value=zeros(4,1)
  year : Constant  Value=epoch.Year
  Modified Julian Date (day) : Outport  VectorParamsAs1DForOutWhenUnconnected=off
  wires:
  Rounding Function/1 -> Sum/2
  If/2 -> If Action Subsystem1/Action
  Gain4/1 -> Sum5/2
  BiasYear/1 -> Gain/1
  Bias2/1 -> Sum1/1
  Selector1/1 -> Sum6/1
  Sum/1 -> Bias2/1
  Sum2/1 -> Sum3/1
  BiasDay/1 -> Sum5/1
  Selector/1 -> Sum3/2
  Sum1/1 -> Sum2/1
  year/1 -> If Action Subsystem1/1, If Action Subsystem/1
  Sum5/1 -> Modified Julian Date (day)/1
  Sum6/1 -> Gain4/1
  hour/1 -> Mux/2
  Gain/1 -> Rounding Function2/1
  Merge1/1 -> Bias1/1
  Since Epoch (sec)/1 -> Assignment/2
  Gain6/1 -> Sum6/3
  Gain2/1 -> Rounding Function1/1
  Mux/1 -> Sum4/1
  Rounding Function1/1 -> Sum1/2, Gain3/1
  Rounding Function3/1 -> Sum2/2
  Sum3/1 -> BiasDay/1
  Selector3/1 -> Gain6/1
  Rounding Function2/1 -> Sum/1
  Gain1/1 -> Rounding Function/1
  sec2/1 -> Assignment/1
  day/1 -> Mux/1
  Bias1/1 -> Gain1/1
  min/1 -> Mux/3
  Gain3/1 -> Rounding Function3/1
  If/1 -> If Action Subsystem/Action
  Gain5/1 -> Sum6/2
  If Action Subsystem1/1 -> Merge/2
  Sum4/1 -> Selector/1, Selector3/1, Selector2/1, Selector1/1
  Merge/1 -> BiasYear/1, Gain2/1
  If Action Subsystem/1 -> Merge/1
  Selector2/1 -> Gain5/1
  If Action Subsystem/2 -> Merge1/1
  month/1 -> If/1, If Action Subsystem1/2, If Action Subsystem/2
  sec/1 -> Mux/4
  If Action Subsystem1/2 -> Merge1/2
  Assignment/1 -> Sum4/2
  Index/1 -> Assignment/3

== system ADCS_MIL/Sensors/GNSS Receiver Model ==
  Calendar : Inport
  Satellite Ephemeris : Inport  Port=2
  " Input Voltage (V)" : Inport  Port=3
  Sensor Switch : Inport  Port=4
  Bus Selector1 : BusSelector  OutputSignals=Julian Date (day)
  Bus Selector7 : BusSelector  OutputSignals=Satellite Velocity [ICRF](m/s),Satellite Position [ICRF](m)
  Gain2 : Gain  Gain=1/(satellite.Gyro.NominalVoltage^2/satellite.Gyro.NominalPower)
  Measured Eph. Bus Creator : BusCreator  Inputs=3
  Mux3 : Mux  Inputs=3
  Mux4 : Mux  Inputs=3
  Product{1..3,5,8} (5 alike) : Product
  Random Noise10 : RandomNumber  Mean=satellite.GPS.Position.Bias  Variance=satellite.GPS.Position.NoiseSTDDEV^2  SampleTime=1/satellite.GPS.Frequency
  Random Noise11 : RandomNumber  Mean=satellite.GPS.Position.Bias  Variance=satellite.GPS.Position.NoiseSTDDEV^2  SampleTime=1/satellite.GPS.Frequency
  Random Noise12 : RandomNumber  Mean=satellite.GPS.Velocity.Bias  Variance=satellite.GPS.Position.NoiseSTDDEV^2  SampleTime=1/satellite.GPS.Frequency
  Random Noise13 : RandomNumber  Mean=satellite.GPS.Velocity.Bias  Variance=satellite.GPS.Position.NoiseSTDDEV^2  SampleTime=1/satellite.GPS.Frequency
  Random Noise14 : RandomNumber  Mean=satellite.GPS.Velocity.Bias  Variance=satellite.GPS.Position.NoiseSTDDEV^2  SampleTime=1/satellite.GPS.Frequency
  Random Noise9 : RandomNumber  Mean=satellite.GPS.Position.Bias  Variance=satellite.GPS.Position.NoiseSTDDEV^2  SampleTime=1/satellite.GPS.Frequency
  Sum2 : Sum  Inputs=|++
  Sum8 : Sum  Inputs=|++
  Unit Delay1 : UnitDelay  SampleTime=-1  HasFrameUpgradeWarning=on
  Zero-Order Hold2 : ZeroOrderHold  SampleTime=1/satellite.GPS.Frequency
  Zero-Order Hold3 : ZeroOrderHold  SampleTime=1/satellite.GPS.Frequency
  Zero-Order Hold4 : ZeroOrderHold  SampleTime=1/satellite.GPS.Frequency
  Measured Satellite Ephemeris : Outport
  Power (W) : Outport  Port=2
  wires:
  Product1/1 -> Measured Eph. Bus Creator/1  "Julian Date (day)"
  Random Noise12/1 -> Mux4/2
  Sum8/1 -> Zero-Order Hold4/1  "Measured Velocity [ITRF] (m/s)"
  Sensor Switch/1 -> Unit Delay1/1
  Zero-Order Hold3/1 -> Product2/1
  Product8/1 -> Measured Eph. Bus Creator/3  "Measured Velocity [ICRF] (m/s)"
  Measured Eph. Bus Creator/1 -> Measured Satellite Ephemeris/1  "Measured Ephemeris"
  Zero-Order Hold2/1 -> Product1/1
  Unit Delay1/1 -> Product1/2, Product2/2, Product8/2, Product5/1
  Product2/1 -> Measured Eph. Bus Creator/2  "Measured Position [ICRF] (m)"
  Product3/1 -> Product5/2
  Product5/1 -> Power (W)/1  "GPS Power Consumption"
  Random Noise9/1 -> Mux3/1
  Bus Selector7/2 -> Sum8/1  "<Satellite Position [ICRF](m)>"
  Zero-Order Hold4/1 -> Product8/1
  Bus Selector7/1 -> Sum2/1  "<Satellite Velocity [ICRF](m/s)>"
  " Input Voltage (V)"/1 -> Gain2/1, Product3/2  "Voltage (V)"
  Sum2/1 -> Zero-Order Hold3/1  "Measured Position [ITRF] (m)"
  Mux3/1 -> Sum2/2
  Random Noise10/1 -> Mux3/2
  Mux4/1 -> Sum8/2
  Random Noise11/1 -> Mux3/3
  Random Noise13/1 -> Mux4/3
  Bus Selector1/1 -> Zero-Order Hold2/1  "<Julian Date (day)>"
  Satellite Ephemeris/1 -> Bus Selector7/1
  Calendar/1 -> Bus Selector1/1
  Gain2/1 -> Product3/1  "Current (A)"
  Random Noise14/1 -> Mux4/1

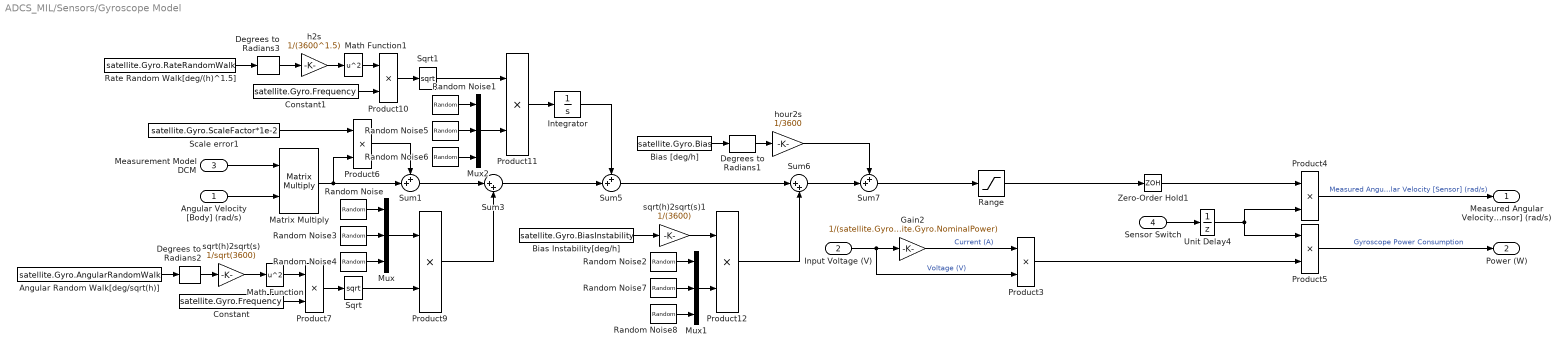
== system ADCS_MIL/Sensors/Gyroscope Model ==
  Angular Velocity [Body] (rad/s) : Inport
  Input Voltage (V) : Inport  Port=2
  Measurement Model DCM : Inport  Port=3
  Sensor Switch : Inport  Port=4
  Angular Random Walk[deg/sqrt(h)] : Constant  Value=satellite.Gyro.AngularRandomWalk
  Bias Instability[deg/h] : Constant  Value=satellite.Gyro.BiasInstability
  Bias [deg/h] : Constant  Value=satellite.Gyro.Bias
  Constant : Constant  Value=satellite.Gyro.Frequency
  Constant1 : Constant  Value=satellite.Gyro.Frequency
  Degrees to Radians1 : simulink_extras/Transformations/Degrees to Radians
  Degrees to Radians2 : simulink_extras/Transformations/Degrees to Radians
  Degrees to Radians3 : simulink_extras/Transformations/Degrees to Radians
  Gain2 : Gain  Gain=1/(satellite.Gyro.NominalVoltage^2/satellite.Gyro.NominalPower)
  Integrator : Integrator  InitialCondition=[0;0;0]
  Math Function : Math  Operator=square  SignedPower=on
  Math Function1 : Math  Operator=square  SignedPower=on
  Matrix Multiply : Product  Multiplication=Matrix(*)
  Mux : Mux  Inputs=3
  Mux1 : Mux  Inputs=3
  Mux2 : Mux  Inputs=3
  Product{3..7,9..12} (9 alike) : Product
  Random Noise{,1..8} (9 alike) : RandomNumber  SampleTime=1/satellite.Gyro.Frequency
  Range : Saturate  UpperLimit=satellite.Gyro.Range(2)  LowerLimit=satellite.Gyro.Range(1)
  Rate Random Walk[deg/(h)^1.5] : Constant  Value=satellite.Gyro.RateRandomWalk
  Scale error1 : Constant  Value=satellite.Gyro.ScaleFactor*1e-2
  Sqrt : Sqrt
  Sqrt1 : Sqrt
  Sum1 : Sum  Inputs=++|
  Sum3 : Sum  Inputs=|++
  Sum5 : Sum  Inputs=++|
  Sum6 : Sum  Inputs=|++
  Sum7 : Sum  Inputs=++|
  Unit Delay4 : UnitDelay  SampleTime=-1  HasFrameUpgradeWarning=on
  Zero-Order Hold1 : ZeroOrderHold  SampleTime=1/satellite.Gyro.Frequency
  h2s : Gain  Gain=1/(3600^1.5)
  hour2s : Gain  Gain=1/3600
  sqrt(h)2sqrt(s) : Gain  Gain=1/sqrt(3600)
  sqrt(h)2sqrt(s)1 : Gain  Gain=1/(3600)
  Measured Angular Velocity [Sensor] (rad/s) : Outport  PortDimensions=[3,1]
  Power (W) : Outport  Port=2
  wires:
  Sqrt/1 -> Product9/2
  Sum1/1 -> Sum3/1
  Sum6/1 -> Sum7/2
  hour2s/1 -> Sum7/1
  Matrix Multiply/1 -> Product6/2, Sum1/2
  Range/1 -> Zero-Order Hold1/1
  Random Noise3/1 -> Mux/2
  Mux/1 -> Product9/1
  Degrees to Radians3/1 -> h2s/1
  Product12/1 -> Sum6/2
  Product9/1 -> Sum3/2
  Product10/1 -> Sqrt1/1
  Random Noise5/1 -> Mux2/2
  Sum5/1 -> Sum6/1
  Integrator/1 -> Sum5/1
  Random Noise6/1 -> Mux2/3
  Math Function/1 -> Product7/1
  Random Noise7/1 -> Mux1/2
  sqrt(h)2sqrt(s)/1 -> Math Function/1
  Mux2/1 -> Product11/2
  Sum7/1 -> Range/1
  Angular Velocity [Body] (rad/s)/1 -> Matrix Multiply/2
  Product3/1 -> Product5/2
  Random Noise2/1 -> Mux1/1
  Constant/1 -> Product7/2
  Bias Instability[deg/h]/1 -> sqrt(h)2sqrt(s)1/1
  Random Noise4/1 -> Mux/3
  Angular Random Walk[deg/sqrt(h)]/1 -> Degrees to Radians2/1
  Gain2/1 -> Product3/1  "Current (A)"
  Random Noise/1 -> Mux/1
  Rate Random Walk[deg/(h)^1.5]/1 -> Degrees to Radians3/1
  Measurement Model DCM/1 -> Matrix Multiply/1
  Product6/1 -> Sum1/1
  Math Function1/1 -> Product10/1
  h2s/1 -> Math Function1/1
  Constant1/1 -> Product10/2
  Product7/1 -> Sqrt/1
  Scale error1/1 -> Product6/1
  Zero-Order Hold1/1 -> Product4/1
  Mux1/1 -> Product12/2
  Sqrt1/1 -> Product11/1
  Product11/1 -> Integrator/1
  Sum3/1 -> Sum5/2
  Sensor Switch/1 -> Unit Delay4/1
  sqrt(h)2sqrt(s)1/1 -> Product12/1
  Bias [deg/h]/1 -> Degrees to Radians1/1
  Degrees to Radians2/1 -> sqrt(h)2sqrt(s)/1
  Product4/1 -> Measured Angular Velocity [Sensor] (rad/s)/1  "Measured Angular Velocity [Sensor] (rad/s)"
  Degrees to Radians1/1 -> hour2s/1
  Random Noise1/1 -> Mux2/1
  Input Voltage (V)/1 -> Product3/2, Gain2/1  "Voltage (V)"
  Unit Delay4/1 -> Product5/1, Product4/2
  Product5/1 -> Power (W)/1  "Gyroscope Power Consumption"
  Random Noise8/1 -> Mux1/3

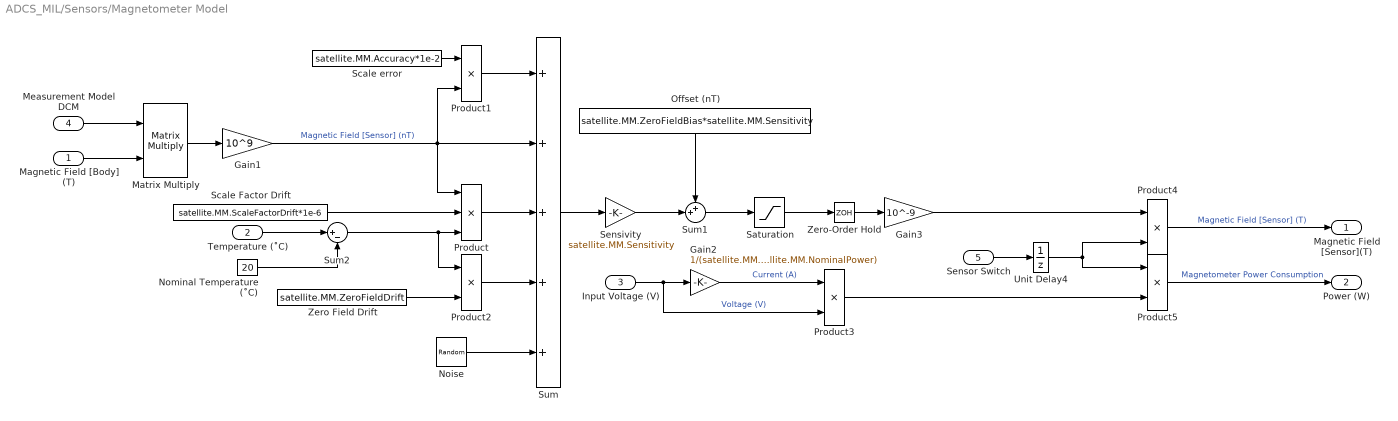
== system ADCS_MIL/Sensors/Magnetometer Model ==
  Magnetic Field [Body] (T) : Inport
  Temperature (˚C) : Inport  Port=2
  Input Voltage (V) : Inport  Port=3
  Measurement Model DCM : Inport  Port=4
  Sensor Switch : Inport  Port=5
  Gain1 : Gain  Gain=10^9
  Gain2 : Gain  Gain=1/(satellite.MM.NominalVoltage^2/satellite.MM.NominalPower)
  Gain3 : Gain  Gain=10^-9
  Matrix Multiply : Product  Multiplication=Matrix(*)
  Noise : RandomNumber  Variance=satellite.MM.NoiseVariance  SampleTime=1/satellite.MM.Frequency
  Nominal Temperature (˚C) : Constant  Value=20
  Offset (nT) : Constant  Value=satellite.MM.ZeroFieldBias*satellite.MM.Sensitivity
  Product : Product  Inputs=3
  Product{1..5} (5 alike) : Product
  Saturation : Saturate  UpperLimit=satellite.MM.Range(2)  LowerLimit=satellite.MM.Range(1)
  Scale Factor Drift : Constant  Value=satellite.MM.ScaleFactorDrift*1e-6
  Scale error : Constant  Value=satellite.MM.Accuracy*1e-2
  Sensivity : Gain  Gain=satellite.MM.Sensitivity
  Sum : Sum  Inputs=+++++
  Sum1 : Sum  Inputs=++|
  Sum2 : Sum  Inputs=|+-
  Unit Delay4 : UnitDelay  SampleTime=-1  HasFrameUpgradeWarning=on
  Zero Field Drift : Constant  Value=satellite.MM.ZeroFieldDrift
  Zero-Order Hold : ZeroOrderHold  SampleTime=1/satellite.MM.Frequency
  Magnetic Field [Sensor](T) : Outport  PortDimensions=[3,1]
  Power (W) : Outport  Port=2
  wires:
  Product3/1 -> Product5/2
  Scale error/1 -> Product1/1
  Sum2/1 -> Product/3, Product2/1
  Saturation/1 -> Zero-Order Hold/1
  Product2/1 -> Sum/4
  Zero-Order Hold/1 -> Gain3/1
  Nominal Temperature (˚C)/1 -> Sum2/2
  Gain2/1 -> Product3/1  "Current (A)"
  Offset (nT)/1 -> Sum1/1
  Measurement Model DCM/1 -> Matrix Multiply/1
  Temperature (˚C)/1 -> Sum2/1
  Product/1 -> Sum/3
  Product1/1 -> Sum/1
  Sensor Switch/1 -> Unit Delay4/1
  Input Voltage (V)/1 -> Gain2/1, Product3/2  "Voltage (V)"
  Sum/1 -> Sensivity/1
  Zero Field Drift/1 -> Product2/2
  Product4/1 -> Magnetic Field [Sensor](T)/1  "Magnetic Field [Sensor] (T)"
  Scale Factor Drift/1 -> Product/2
  Noise/1 -> Sum/5
  Gain1/1 -> Product1/2, Product/1, Sum/2  "Magnetic Field [Sensor] (nT)"
  Sum1/1 -> Saturation/1
  Sensivity/1 -> Sum1/2
  Magnetic Field [Body] (T)/1 -> Matrix Multiply/2
  Gain3/1 -> Product4/1
  Unit Delay4/1 -> Product4/2, Product5/1
  Matrix Multiply/1 -> Gain1/1
  Product5/1 -> Power (W)/1  "Magnetometer Power Consumption"
